simulink model "bh_DBL_CONTROL"  (R2016a)
settings: Solver=ode15s  StartTime=0.0  StopTime=30  FixedStep=0.01  RelTol=1e-5
undefined symbols (not defined in the file or in its folder): b1_damp, b2_damp, g, I1g, I2g, L1x, L2x, mass1, mass2
libraries: simulink x5
settings Model: Creator=bhorton  LastModifiedBy=bhorton
settings SolverCC: ZeroCrossAlgorithm=Adaptive
settings GRTTargetCC: GeneratePreprocessorConditionals=Use local settings
settings SimscapeCC: SimscapeLogType=all  SimscapeLogDataHistory=10000  SelectedTab=Simscape Multibody

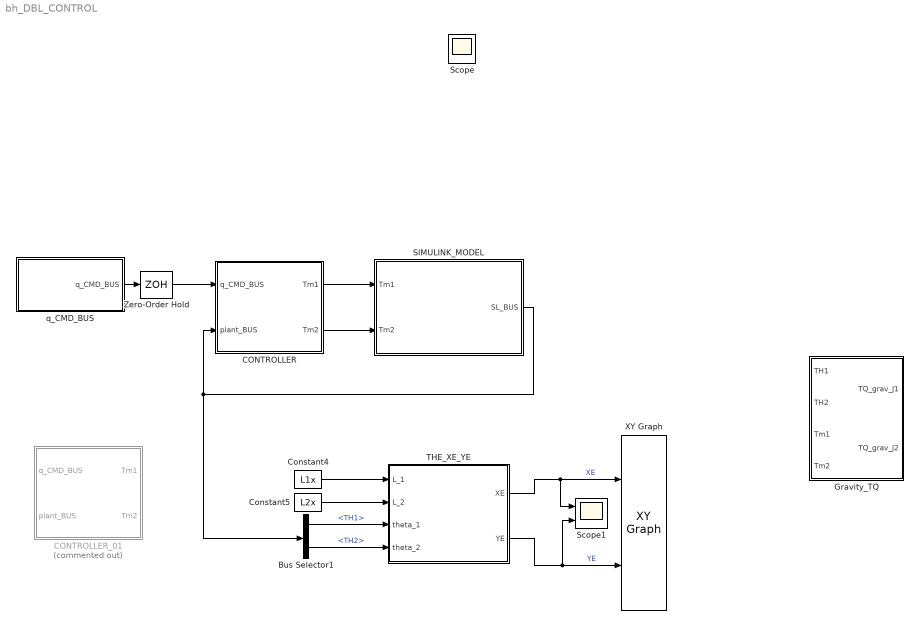
== system bh_DBL_CONTROL ==
  Bus Selector1 : BusSelector  OutputSignals=TH1,TH2
  CONTROLLER : Subsystem
  CONTROLLER_01 : Subsystem  Commented=on
  Constant4 : Constant  Value=L1x
  Constant5 : Constant  Value=L2x
  Gravity_TQ : Subsystem
  SIMULINK_MODEL : Subsystem
  Scope1 : Scope  NumInputPorts=2
  THE_XE_YE : MATLAB Function  TreatAsAtomicUnit=on
  XY Graph : simulink/Sinks/XY Graph  xmin=0  xmax=1.6  ymin=0  ymax=1.6  st=-1
  Zero-Order Hold : ZeroOrderHold  SampleTime=0.01
  q_CMD_BUS : Subsystem
  Scope : Scope
  wires:
  SIMULINK_MODEL/1(SL_BUS) -> CONTROLLER/2(plant_BUS), Bus Selector1/1
  CONTROLLER/1(Tm1) -> SIMULINK_MODEL/1(Tm1)
  CONTROLLER/2(Tm2) -> SIMULINK_MODEL/2(Tm2)
  q_CMD_BUS/1(q_CMD_BUS) -> Zero-Order Hold/1
  Constant5/1 -> THE_XE_YE/2(L_2)
  Constant4/1 -> THE_XE_YE/1(L_1)
  THE_XE_YE/1(XE) -> Scope1/1, XY Graph/1  "XE"
  THE_XE_YE/2(YE) -> Scope1/2, XY Graph/2  "YE"
  Bus Selector1/1 -> THE_XE_YE/3(theta_1)  "<TH1>"
  Bus Selector1/2 -> THE_XE_YE/4(theta_2)  "<TH2>"
  Zero-Order Hold/1 -> CONTROLLER/1(q_CMD_BUS)

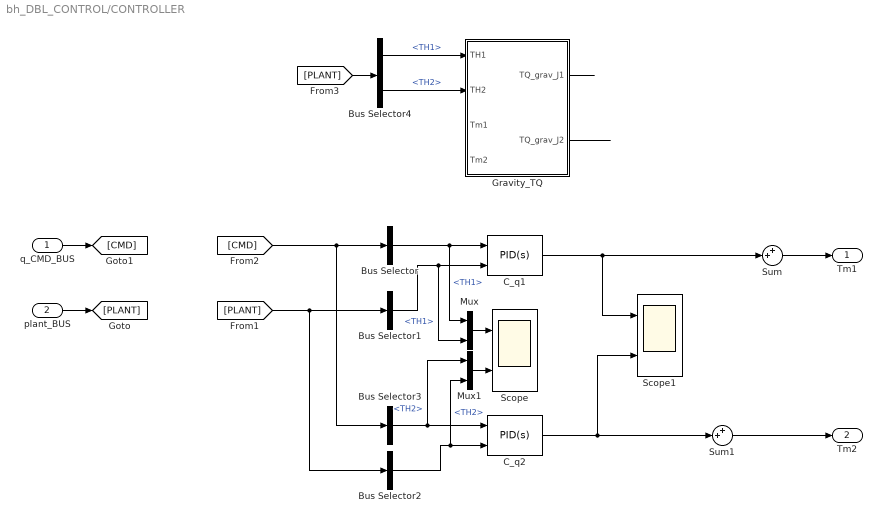
== system bh_DBL_CONTROL/CONTROLLER ==
  q_CMD_BUS : Inport
  plant_BUS : Inport  Port=2
  Bus Selector : BusSelector  OutputSignals=TH1
  Bus Selector1 : BusSelector  OutputSignals=TH1
  Bus Selector2 : BusSelector  OutputSignals=TH2
  Bus Selector3 : BusSelector  OutputSignals=TH2
  Bus Selector4 : BusSelector  OutputSignals=TH1,TH2
  C_q1 : simulink/Continuous/PID Controller (2DOF)  Controller=PID  TimeDomain=Continuous-time  SampleTime=-1  IntegratorMethod=Forward Euler  FilterMethod=Forward Euler  Form=Parallel  UseFilter=on  ControllerParametersSource=internal  P=1357.56511671981  I=4845.84125529163  D=84.5236806608288  N=69907.371435519  b=0.974411131828766  c=0.922736671022408  InitialConditionSource=internal  InitialConditionForIntegrator=0  InitialConditionForFilter=0  ExternalReset=none  LimitOutput=off  UpperSaturationLimit=inf  LowerSaturationLimit=-inf  LinearizeAsGain=on  AntiWindupMode=none  Kb=1  TrackingMode=off  Kt=1  PParamMin=[]  PParamMax=[]  IParamMin=[]  IParamMax=[]  DParamMin=[]  DParamMax=[]  NParamMin=[]  NParamMax=[]  bParamMin=[]  bParamMax=[]  cParamMin=[]  cParamMax=[]  KbParamMin=[]  KbParamMax=[]  KtParamMin=[]  KtParamMax=[]  POutMin=[]  POutMax=[]  IOutMin=[]  IOutMax=[]  DOutMin=[]  DOutMax=[]  NOutMin=[]  NOutMax=[]  bOutMin=[]  bOutMax=[]  cOutMin=[]  cOutMax=[]  KbOutMin=[]  KbOutMax=[]  KtOutMin=[]  KtOutMax=[]  IntegratorOutMin=[]  IntegratorOutMax=[]  FilterOutMin=[]  FilterOutMax=[]  SumOutMin=[]  SumOutMax=[]  Sum1OutMin=[]  Sum1OutMax=[]  Sum2OutMin=[]  Sum2OutMax=[]  Sum3OutMin=[]  Sum3OutMax=[]  SumI1OutMin=[]  SumI1OutMax=[]  SumI2OutMin=[]  SumI2OutMax=[]  SumI3OutMin=[]  SumI3OutMax=[]  SumDOutMin=[]  SumDOutMax=[]  SaturationOutMin=[]  SaturationOutMax=[]  IntegratorContinuousStateAttributes=''  IntegratorStateMustResolveToSignalObject=off  IntegratorRTWStateStorageClass=Auto  FilterContinuousStateAttributes=''  FilterStateMustResolveToSignalObject=off  FilterRTWStateStorageClass=Auto  DifferentiatorICPrevScaledInput=0  DifferentiatorOutMin=[]  DifferentiatorOutMax=[]
  C_q2 : simulink/Continuous/PID Controller (2DOF)  Controller=PID  TimeDomain=Continuous-time  SampleTime=-1  IntegratorMethod=Forward Euler  FilterMethod=Forward Euler  Form=Parallel  UseFilter=on  ControllerParametersSource=internal  P=8716881.64195116  I=38875375820.2039  D=480.022145350049  N=516158.444640812  b=1.01267061686983  c=0.794786207270043  InitialConditionSource=internal  InitialConditionForIntegrator=0  InitialConditionForFilter=0  ExternalReset=none  LimitOutput=off  UpperSaturationLimit=inf  LowerSaturationLimit=-inf  LinearizeAsGain=on  AntiWindupMode=none  Kb=1  TrackingMode=off  Kt=1  PParamMin=[]  PParamMax=[]  IParamMin=[]  IParamMax=[]  DParamMin=[]  DParamMax=[]  NParamMin=[]  NParamMax=[]  bParamMin=[]  bParamMax=[]  cParamMin=[]  cParamMax=[]  KbParamMin=[]  KbParamMax=[]  KtParamMin=[]  KtParamMax=[]  POutMin=[]  POutMax=[]  IOutMin=[]  IOutMax=[]  DOutMin=[]  DOutMax=[]  NOutMin=[]  NOutMax=[]  bOutMin=[]  bOutMax=[]  cOutMin=[]  cOutMax=[]  KbOutMin=[]  KbOutMax=[]  KtOutMin=[]  KtOutMax=[]  IntegratorOutMin=[]  IntegratorOutMax=[]  FilterOutMin=[]  FilterOutMax=[]  SumOutMin=[]  SumOutMax=[]  Sum1OutMin=[]  Sum1OutMax=[]  Sum2OutMin=[]  Sum2OutMax=[]  Sum3OutMin=[]  Sum3OutMax=[]  SumI1OutMin=[]  SumI1OutMax=[]  SumI2OutMin=[]  SumI2OutMax=[]  SumI3OutMin=[]  SumI3OutMax=[]  SumDOutMin=[]  SumDOutMax=[]  SaturationOutMin=[]  SaturationOutMax=[]  IntegratorContinuousStateAttributes=''  IntegratorStateMustResolveToSignalObject=off  IntegratorRTWStateStorageClass=Auto  FilterContinuousStateAttributes=''  FilterStateMustResolveToSignalObject=off  FilterRTWStateStorageClass=Auto  DifferentiatorICPrevScaledInput=0  DifferentiatorOutMin=[]  DifferentiatorOutMax=[]
  Gravity_TQ : Subsystem
  Mux : Mux  Inputs=2
  Mux1 : Mux  Inputs=2
  Scope : Scope  NumInputPorts=2
  Scope1 : Scope  NumInputPorts=2
  Sum : Sum  Inputs=++|
  Sum1 : Sum  Inputs=++|
  Tm1 : Outport
  Tm2 : Outport  Port=2
  wires:
  [CMD] -> Bus Selector3/1, Bus Selector/1
  [PLANT] -> Bus Selector2/1, Bus Selector1/1
  Bus Selector/1 -> Mux/1, C_q1/1  "<TH1>"
  Bus Selector1/1 -> Mux/2, C_q1/2  "<TH1>"
  Bus Selector3/1 -> Mux1/1, C_q2/1  "<TH2>"
  Bus Selector2/1 -> C_q2/2, Mux1/2  "<TH2>"
  Mux/1 -> Scope/1
  Mux1/1 -> Scope/2
  plant_BUS/1 -> [PLANT]
  q_CMD_BUS/1 -> [CMD]
  [PLANT] -> Bus Selector4/1
  Bus Selector4/1 -> Gravity_TQ/1(TH1)  "<TH1>"
  Bus Selector4/2 -> Gravity_TQ/2(TH2)  "<TH2>"
  Sum/1 -> Tm1/1
  C_q1/1 -> Scope1/1, Sum/2
  Gravity_TQ/1(TQ_grav_J1) -> ?
  Gravity_TQ/2(TQ_grav_J2) -> ?
  Sum1/1 -> Tm2/1
  C_q2/1 -> Scope1/2, Sum1/2

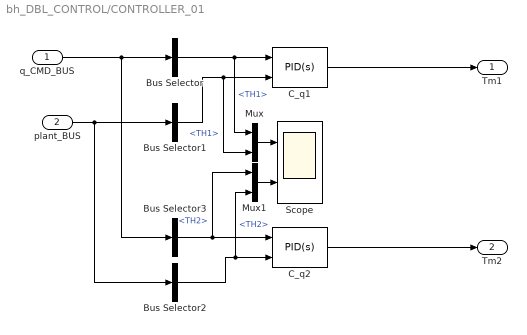
== system bh_DBL_CONTROL/CONTROLLER_01 ==
  q_CMD_BUS : Inport
  plant_BUS : Inport  Port=2
  Bus Selector : BusSelector  OutputSignals=TH1
  Bus Selector1 : BusSelector  OutputSignals=TH1
  Bus Selector2 : BusSelector  OutputSignals=TH2
  Bus Selector3 : BusSelector  OutputSignals=TH2
  C_q1 : simulink/Continuous/PID Controller (2DOF)  Controller=PID  TimeDomain=Continuous-time  SampleTime=-1  IntegratorMethod=Forward Euler  FilterMethod=Forward Euler  Form=Parallel  UseFilter=on  ControllerParametersSource=internal  P=1357.56511671981  I=4845.84125529163  D=84.5236806608288  N=69907.371435519  b=0.974411131828766  c=0.922736671022408  InitialConditionSource=internal  InitialConditionForIntegrator=0  InitialConditionForFilter=0  ExternalReset=none  LimitOutput=off  UpperSaturationLimit=inf  LowerSaturationLimit=-inf  LinearizeAsGain=on  AntiWindupMode=none  Kb=1  TrackingMode=off  Kt=1  PParamMin=[]  PParamMax=[]  IParamMin=[]  IParamMax=[]  DParamMin=[]  DParamMax=[]  NParamMin=[]  NParamMax=[]  bParamMin=[]  bParamMax=[]  cParamMin=[]  cParamMax=[]  KbParamMin=[]  KbParamMax=[]  KtParamMin=[]  KtParamMax=[]  POutMin=[]  POutMax=[]  IOutMin=[]  IOutMax=[]  DOutMin=[]  DOutMax=[]  NOutMin=[]  NOutMax=[]  bOutMin=[]  bOutMax=[]  cOutMin=[]  cOutMax=[]  KbOutMin=[]  KbOutMax=[]  KtOutMin=[]  KtOutMax=[]  IntegratorOutMin=[]  IntegratorOutMax=[]  FilterOutMin=[]  FilterOutMax=[]  SumOutMin=[]  SumOutMax=[]  Sum1OutMin=[]  Sum1OutMax=[]  Sum2OutMin=[]  Sum2OutMax=[]  Sum3OutMin=[]  Sum3OutMax=[]  SumI1OutMin=[]  SumI1OutMax=[]  SumI2OutMin=[]  SumI2OutMax=[]  SumI3OutMin=[]  SumI3OutMax=[]  SumDOutMin=[]  SumDOutMax=[]  SaturationOutMin=[]  SaturationOutMax=[]  IntegratorContinuousStateAttributes=''  IntegratorStateMustResolveToSignalObject=off  IntegratorRTWStateStorageClass=Auto  FilterContinuousStateAttributes=''  FilterStateMustResolveToSignalObject=off  FilterRTWStateStorageClass=Auto  DifferentiatorICPrevScaledInput=0  DifferentiatorOutMin=[]  DifferentiatorOutMax=[]
  C_q2 : simulink/Continuous/PID Controller (2DOF)  Controller=PID  TimeDomain=Continuous-time  SampleTime=-1  IntegratorMethod=Forward Euler  FilterMethod=Forward Euler  Form=Parallel  UseFilter=on  ControllerParametersSource=internal  P=8716881.64195116  I=38875375820.2039  D=480.022145350049  N=516158.444640812  b=1.01267061686983  c=0.794786207270043  InitialConditionSource=internal  InitialConditionForIntegrator=0  InitialConditionForFilter=0  ExternalReset=none  LimitOutput=off  UpperSaturationLimit=inf  LowerSaturationLimit=-inf  LinearizeAsGain=on  AntiWindupMode=none  Kb=1  TrackingMode=off  Kt=1  PParamMin=[]  PParamMax=[]  IParamMin=[]  IParamMax=[]  DParamMin=[]  DParamMax=[]  NParamMin=[]  NParamMax=[]  bParamMin=[]  bParamMax=[]  cParamMin=[]  cParamMax=[]  KbParamMin=[]  KbParamMax=[]  KtParamMin=[]  KtParamMax=[]  POutMin=[]  POutMax=[]  IOutMin=[]  IOutMax=[]  DOutMin=[]  DOutMax=[]  NOutMin=[]  NOutMax=[]  bOutMin=[]  bOutMax=[]  cOutMin=[]  cOutMax=[]  KbOutMin=[]  KbOutMax=[]  KtOutMin=[]  KtOutMax=[]  IntegratorOutMin=[]  IntegratorOutMax=[]  FilterOutMin=[]  FilterOutMax=[]  SumOutMin=[]  SumOutMax=[]  Sum1OutMin=[]  Sum1OutMax=[]  Sum2OutMin=[]  Sum2OutMax=[]  Sum3OutMin=[]  Sum3OutMax=[]  SumI1OutMin=[]  SumI1OutMax=[]  SumI2OutMin=[]  SumI2OutMax=[]  SumI3OutMin=[]  SumI3OutMax=[]  SumDOutMin=[]  SumDOutMax=[]  SaturationOutMin=[]  SaturationOutMax=[]  IntegratorContinuousStateAttributes=''  IntegratorStateMustResolveToSignalObject=off  IntegratorRTWStateStorageClass=Auto  FilterContinuousStateAttributes=''  FilterStateMustResolveToSignalObject=off  FilterRTWStateStorageClass=Auto  DifferentiatorICPrevScaledInput=0  DifferentiatorOutMin=[]  DifferentiatorOutMax=[]
  Mux : Mux  Inputs=2
  Mux1 : Mux  Inputs=2
  Scope : Scope  NumInputPorts=2
  Tm1 : Outport
  Tm2 : Outport  Port=2
  wires:
  q_CMD_BUS/1 -> Bus Selector3/1, Bus Selector/1
  plant_BUS/1 -> Bus Selector2/1, Bus Selector1/1
  Bus Selector/1 -> Mux/1, C_q1/1  "<TH1>"
  Bus Selector1/1 -> Mux/2, C_q1/2  "<TH1>"
  C_q1/1 -> Tm1/1
  Bus Selector3/1 -> Mux1/1, C_q2/1  "<TH2>"
  Bus Selector2/1 -> C_q2/2, Mux1/2  "<TH2>"
  C_q2/1 -> Tm2/1
  Mux/1 -> Scope/1
  Mux1/1 -> Scope/2

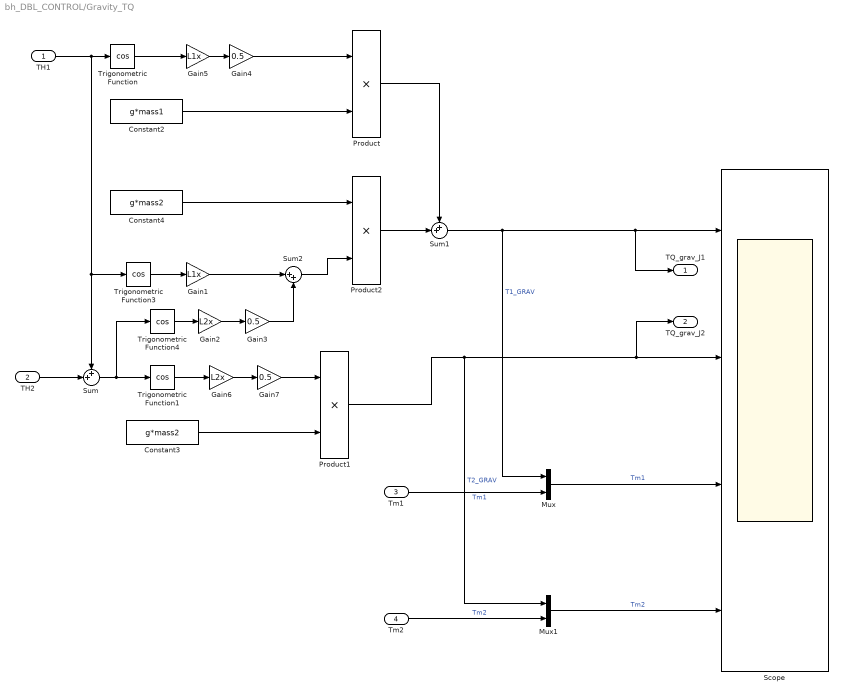
== system bh_DBL_CONTROL/Gravity_TQ ==
  TH1 : Inport
  TH2 : Inport  Port=2
  Tm1 : Inport  Port=3
  Tm2 : Inport  Port=4
  Constant2 : Constant  Value=g*mass1
  Constant3 : Constant  Value=g*mass2
  Constant4 : Constant  Value=g*mass2
  Gain1 : Gain  Gain=L1x
  Gain2 : Gain  Gain=L2x
  Gain3 : Gain  Gain=0.5
  Gain4 : Gain  Gain=0.5
  Gain5 : Gain  Gain=L1x
  Gain6 : Gain  Gain=L2x
  Gain7 : Gain  Gain=0.5
  Mux : Mux  Inputs=2
  Mux1 : Mux  Inputs=2
  Product : Product
  Product1 : Product
  Product2 : Product
  Scope : Scope  NumInputPorts=4
  Sum : Sum  Inputs=++|
  Sum1 : Sum  Inputs=++|
  Sum2 : Sum  Inputs=|++
  Trigonometric Function{,1,3..4} (4 alike) : Trigonometry  Operator=cos
  TQ_grav_J1 : Outport
  TQ_grav_J2 : Outport  Port=2
  wires:
  TH2/1 -> Sum/2
  Sum/1 -> Trigonometric Function4/1, Trigonometric Function1/1
  Trigonometric Function/1 -> Gain5/1
  Trigonometric Function1/1 -> Gain6/1
  Constant3/1 -> Product1/2
  Product/1 -> Sum1/1
  TH1/1 -> Trigonometric Function/1, Trigonometric Function3/1, Sum/1
  Constant2/1 -> Product/2
  Constant4/1 -> Product2/1
  Trigonometric Function3/1 -> Gain1/1
  Gain1/1 -> Sum2/1
  Trigonometric Function4/1 -> Gain2/1
  Gain2/1 -> Gain3/1
  Gain3/1 -> Sum2/2
  Sum2/1 -> Product2/2
  Product2/1 -> Sum1/2
  Sum1/1 -> Mux/1, TQ_grav_J1/1, Scope/1  "T1_GRAV"
  Product1/1 -> Mux1/1, TQ_grav_J2/1, Scope/2  "T2_GRAV"
  Mux/1 -> Scope/3  "Tm1"
  Mux1/1 -> Scope/4  "Tm2"
  Tm1/1 -> Mux/2  "Tm1"
  Tm2/1 -> Mux1/2  "Tm2"
  Gain5/1 -> Gain4/1
  Gain4/1 -> Product/1
  Gain6/1 -> Gain7/1
  Gain7/1 -> Product1/1

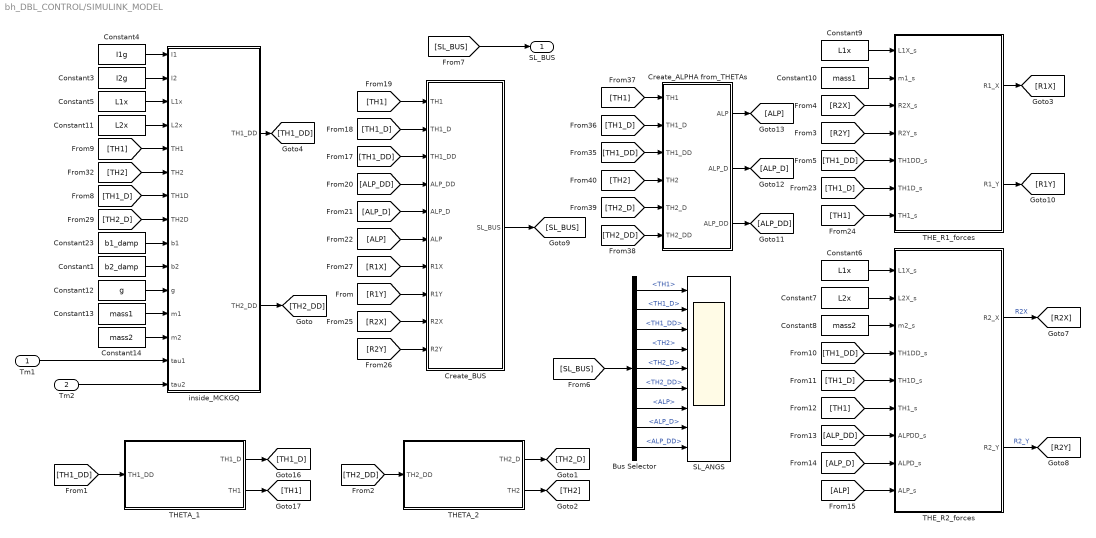
== system bh_DBL_CONTROL/SIMULINK_MODEL ==
  Tm1 : Inport
  Tm2 : Inport  Port=2
  Bus Selector : BusSelector  OutputSignals=TH1,TH1_D,TH1_DD,TH2,TH2_D,TH2_DD,ALP,ALP_D,ALP_DD
  Constant1 : Constant  Value=b2_damp
  Constant10 : Constant  Value=mass1
  Constant11 : Constant  Value=L2x
  Constant12 : Constant  Value=g
  Constant13 : Constant  Value=mass1
  Constant14 : Constant  Value=mass2
  Constant23 : Constant  Value=b1_damp
  Constant3 : Constant  Value=I2g
  Constant4 : Constant  Value=I1g
  Constant5 : Constant  Value=L1x
  Constant6 : Constant  Value=L1x
  Constant7 : Constant  Value=L2x
  Constant8 : Constant  Value=mass2
  Constant9 : Constant  Value=L1x
  Create_ALPHA from_THETAs : Subsystem
  Create_BUS : Subsystem
  SL_ANGS : Scope  NumInputPorts=9
  THETA_1 : Subsystem
  THETA_2 : Subsystem
  THE_R1_forces : MATLAB Function  TreatAsAtomicUnit=on
  THE_R2_forces : MATLAB Function  TreatAsAtomicUnit=on
  inside_MCKGQ : Subsystem
  SL_BUS : Outport
  wires:
  [SL_BUS] -> Bus Selector/1
  [SL_BUS] -> SL_BUS/1
  Constant6/1 -> THE_R2_forces/1(L1X_s)
  Constant7/1 -> THE_R2_forces/2(L2X_s)
  Constant8/1 -> THE_R2_forces/3(m2_s)
  [ALP_DD] -> THE_R2_forces/7(ALPDD_s)
  [ALP_D] -> THE_R2_forces/8(ALPD_s)
  [ALP] -> THE_R2_forces/9(ALP_s)
  [TH1] -> THE_R2_forces/6(TH1_s)
  [TH1_D] -> THE_R2_forces/5(TH1D_s)
  [TH1_DD] -> THE_R2_forces/4(TH1DD_s)
  THE_R2_forces/2(R2_Y) -> [R2Y]  "R2_Y"
  THE_R2_forces/1(R2_X) -> [R2X]  "R2X"
  [ALP_D] -> Create_BUS/5(ALP_D)
  [TH1_D] -> Create_BUS/2(TH1_D)
  [ALP_DD] -> Create_BUS/4(ALP_DD)
  [ALP] -> Create_BUS/6(ALP)
  [TH1_DD] -> Create_BUS/3(TH1_DD)
  [TH1] -> Create_BUS/1(TH1)
  Create_BUS/1(SL_BUS) -> [SL_BUS]
  Bus Selector/2 -> SL_ANGS/2  "<TH1_D>"
  Bus Selector/3 -> SL_ANGS/3  "<TH1_DD>"
  Bus Selector/1 -> SL_ANGS/1  "<TH1>"
  Bus Selector/4 -> SL_ANGS/4  "<TH2>"
  Bus Selector/5 -> SL_ANGS/5  "<TH2_D>"
  Bus Selector/6 -> SL_ANGS/6  "<TH2_DD>"
  Bus Selector/7 -> SL_ANGS/7  "<ALP>"
  Bus Selector/8 -> SL_ANGS/8  "<ALP_D>"
  Bus Selector/9 -> SL_ANGS/9  "<ALP_DD>"
  Constant9/1 -> THE_R1_forces/1(L1X_s)
  Constant10/1 -> THE_R1_forces/2(m1_s)
  [R2X] -> THE_R1_forces/3(R2X_s)
  [R2Y] -> THE_R1_forces/4(R2Y_s)
  [TH1] -> THE_R1_forces/7(TH1_s)
  [TH1_D] -> THE_R1_forces/6(TH1D_s)
  [TH1_DD] -> THE_R1_forces/5(TH1DD_s)
  THE_R1_forces/2(R1_Y) -> [R1Y]
  THE_R1_forces/1(R1_X) -> [R1X]
  [R1X] -> Create_BUS/7(R1X)
  [R1Y] -> Create_BUS/8(R1Y)
  [R2Y] -> Create_BUS/10(R2Y)
  [R2X] -> Create_BUS/9(R2X)
  Constant4/1 -> inside_MCKGQ/1(I1)
  Constant3/1 -> inside_MCKGQ/2(I2)
  Constant11/1 -> inside_MCKGQ/4(L2x)
  Constant5/1 -> inside_MCKGQ/3(L1x)
  Constant12/1 -> inside_MCKGQ/11(g)
  Constant13/1 -> inside_MCKGQ/12(m1)
  Constant14/1 -> inside_MCKGQ/13(m2)
  [TH1] -> inside_MCKGQ/5(TH1)
  [TH2] -> inside_MCKGQ/6(TH2)
  [TH1_D] -> Create_ALPHA from_THETAs/2(TH1_D)
  [TH1_DD] -> Create_ALPHA from_THETAs/3(TH1_DD)
  [TH1] -> Create_ALPHA from_THETAs/1(TH1)
  [TH2] -> Create_ALPHA from_THETAs/4(TH2)
  [TH2_D] -> Create_ALPHA from_THETAs/5(TH2_D)
  [TH2_DD] -> Create_ALPHA from_THETAs/6(TH2_DD)
  Create_ALPHA from_THETAs/2(ALP_D) -> [ALP_D]
  Create_ALPHA from_THETAs/3(ALP_DD) -> [ALP_DD]
  Create_ALPHA from_THETAs/1(ALP) -> [ALP]
  [TH1_D] -> inside_MCKGQ/7(TH1D)
  [TH2_D] -> inside_MCKGQ/8(TH2D)
  [TH2_DD] -> THETA_2/1(TH2_DD)
  THETA_2/2(TH2) -> [TH2]
  THETA_2/1(TH2_D) -> [TH2_D]
  [TH1_DD] -> THETA_1/1(TH1_DD)
  THETA_1/1(TH1_D) -> [TH1_D]
  THETA_1/2(TH1) -> [TH1]
  Constant23/1 -> inside_MCKGQ/9(b1)
  Constant1/1 -> inside_MCKGQ/10(b2)
  inside_MCKGQ/1(TH1_DD) -> [TH1_DD]
  inside_MCKGQ/2(TH2_DD) -> [TH2_DD]
  Tm1/1 -> inside_MCKGQ/14(tau1)
  Tm2/1 -> inside_MCKGQ/15(tau2)

== system bh_DBL_CONTROL/q_CMD_BUS ==
  Bus Creator : BusCreator  Inputs=4
  Bus Selector : BusSelector  OutputSignals=TH1_DOT,TH2_DOT,TH1,TH2
  From Spreadsheet : FromSpreadsheet  FileName=bh_2dof_q1_q2_for_hello.xlsx  SheetName=Q_for_hello  SampleTime=-1  ExtrapolationBeforeFirstDataPoint=Hold first value  ExtrapolationAfterLastDataPoint=Hold last value
  Scope : Scope  NumInputPorts=4
  q_CMD_BUS : Outport
  wires:
  From Spreadsheet/2 -> Bus Creator/2  "TH2_DOT"
  From Spreadsheet/3 -> Bus Creator/3  "TH1"
  From Spreadsheet/1 -> Bus Creator/1  "TH1_DOT"
  From Spreadsheet/4 -> Bus Creator/4  "TH2"
  Bus Creator/1 -> Bus Selector/1, q_CMD_BUS/1
  Bus Selector/1 -> Scope/1  "<TH1_DOT>"
  Bus Selector/2 -> Scope/2  "<TH2_DOT>"
  Bus Selector/3 -> Scope/3  "<TH1>"
  Bus Selector/4 -> Scope/4  "<TH2>"

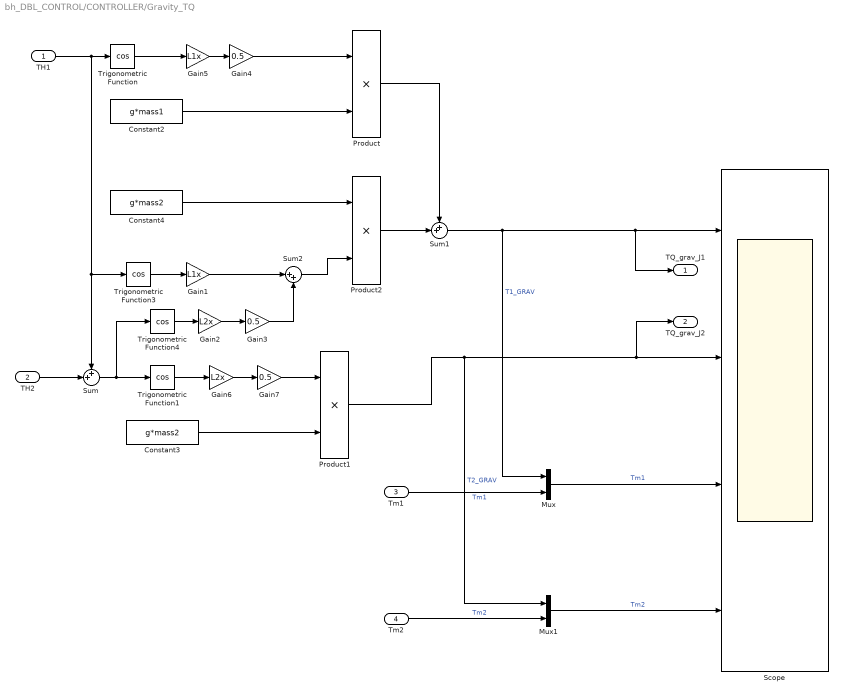
== system bh_DBL_CONTROL/CONTROLLER/Gravity_TQ ==
  TH1 : Inport
  TH2 : Inport  Port=2
  Tm1 : Inport  Port=3
  Tm2 : Inport  Port=4
  Constant2 : Constant  Value=g*mass1
  Constant3 : Constant  Value=g*mass2
  Constant4 : Constant  Value=g*mass2
  Gain1 : Gain  Gain=L1x
  Gain2 : Gain  Gain=L2x
  Gain3 : Gain  Gain=0.5
  Gain4 : Gain  Gain=0.5
  Gain5 : Gain  Gain=L1x
  Gain6 : Gain  Gain=L2x
  Gain7 : Gain  Gain=0.5
  Mux : Mux  Inputs=2
  Mux1 : Mux  Inputs=2
  Product : Product
  Product1 : Product
  Product2 : Product
  Scope : Scope  NumInputPorts=4
  Sum : Sum  Inputs=++|
  Sum1 : Sum  Inputs=++|
  Sum2 : Sum  Inputs=|++
  Trigonometric Function{,1,3..4} (4 alike) : Trigonometry  Operator=cos
  TQ_grav_J1 : Outport
  TQ_grav_J2 : Outport  Port=2
  wires:
  TH2/1 -> Sum/2
  Sum/1 -> Trigonometric Function4/1, Trigonometric Function1/1
  Trigonometric Function/1 -> Gain5/1
  Trigonometric Function1/1 -> Gain6/1
  Constant3/1 -> Product1/2
  Product/1 -> Sum1/1
  TH1/1 -> Trigonometric Function/1, Trigonometric Function3/1, Sum/1
  Constant2/1 -> Product/2
  Constant4/1 -> Product2/1
  Trigonometric Function3/1 -> Gain1/1
  Gain1/1 -> Sum2/1
  Trigonometric Function4/1 -> Gain2/1
  Gain2/1 -> Gain3/1
  Gain3/1 -> Sum2/2
  Sum2/1 -> Product2/2
  Product2/1 -> Sum1/2
  Sum1/1 -> Mux/1, TQ_grav_J1/1, Scope/1  "T1_GRAV"
  Product1/1 -> Mux1/1, TQ_grav_J2/1, Scope/2  "T2_GRAV"
  Mux/1 -> Scope/3  "Tm1"
  Mux1/1 -> Scope/4  "Tm2"
  Tm1/1 -> Mux/2  "Tm1"
  Tm2/1 -> Mux1/2  "Tm2"
  Gain5/1 -> Gain4/1
  Gain4/1 -> Product/1
  Gain6/1 -> Gain7/1
  Gain7/1 -> Product1/1

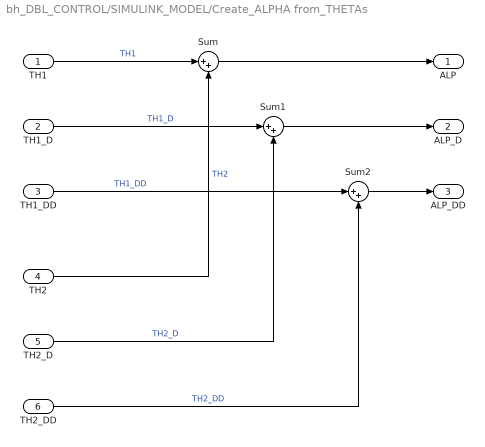
== system bh_DBL_CONTROL/SIMULINK_MODEL/Create_ALPHA from_THETAs ==
  TH1 : Inport
  TH1_D : Inport  Port=2
  TH1_DD : Inport  Port=3
  TH2 : Inport  Port=4
  TH2_D : Inport  Port=5
  TH2_DD : Inport  Port=6
  Sum : Sum  Inputs=|++
  Sum1 : Sum  Inputs=|++
  Sum2 : Sum  Inputs=|++
  ALP : Outport
  ALP_D : Outport  Port=2
  ALP_DD : Outport  Port=3
  wires:
  TH1_DD/1 -> Sum2/1  "TH1_DD"
  TH1_D/1 -> Sum1/1  "TH1_D"
  TH1/1 -> Sum/1  "TH1"
  TH2_DD/1 -> Sum2/2  "TH2_DD"
  TH2_D/1 -> Sum1/2  "TH2_D"
  TH2/1 -> Sum/2  "TH2"
  Sum/1 -> ALP/1
  Sum1/1 -> ALP_D/1
  Sum2/1 -> ALP_DD/1

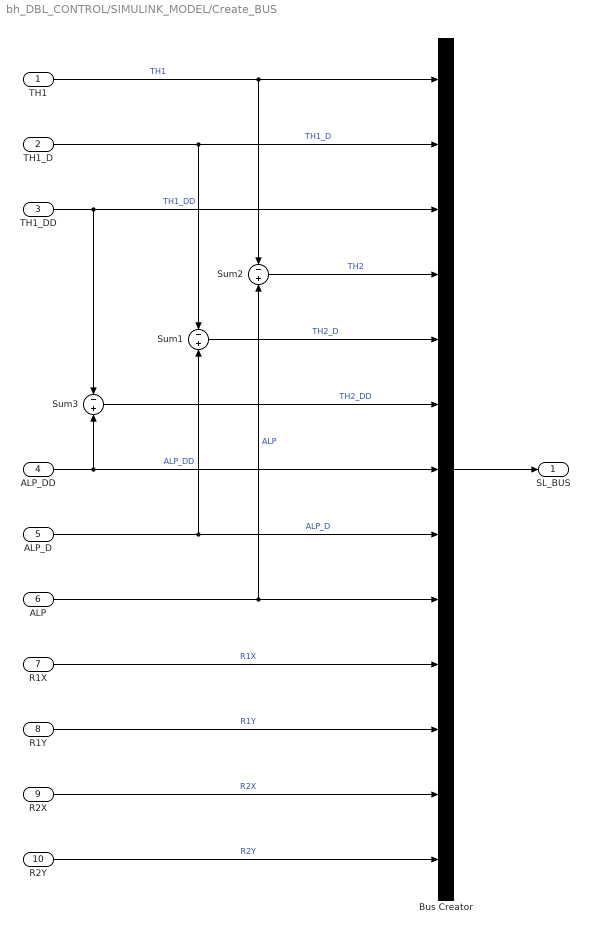
== system bh_DBL_CONTROL/SIMULINK_MODEL/Create_BUS ==
  TH1 : Inport
  TH1_D : Inport  Port=2
  TH1_DD : Inport  Port=3
  ALP_DD : Inport  Port=4
  ALP_D : Inport  Port=5
  ALP : Inport  Port=6
  R1X : Inport  Port=7
  R1Y : Inport  Port=8
  R2X : Inport  Port=9
  R2Y : Inport  Port=10
  Bus Creator : BusCreator  Inputs=13
  Sum1 : Sum  Inputs=-|+
  Sum2 : Sum  Inputs=-|+
  Sum3 : Sum  Inputs=-|+
  SL_BUS : Outport
  wires:
  ALP_DD/1 -> Bus Creator/7, Sum3/2  "ALP_DD"
  TH1_DD/1 -> Sum3/1, Bus Creator/3  "TH1_DD"
  TH1_D/1 -> Bus Creator/2, Sum1/1  "TH1_D"
  ALP_D/1 -> Bus Creator/8, Sum1/2  "ALP_D"
  TH1/1 -> Bus Creator/1, Sum2/1  "TH1"
  ALP/1 -> Bus Creator/9, Sum2/2  "ALP"
  Sum2/1 -> Bus Creator/4  "TH2"
  Sum1/1 -> Bus Creator/5  "TH2_D"
  Sum3/1 -> Bus Creator/6  "TH2_DD"
  Bus Creator/1 -> SL_BUS/1
  R1Y/1 -> Bus Creator/11  "R1Y"
  R1X/1 -> Bus Creator/10  "R1X"
  R2Y/1 -> Bus Creator/13  "R2Y"
  R2X/1 -> Bus Creator/12  "R2X"

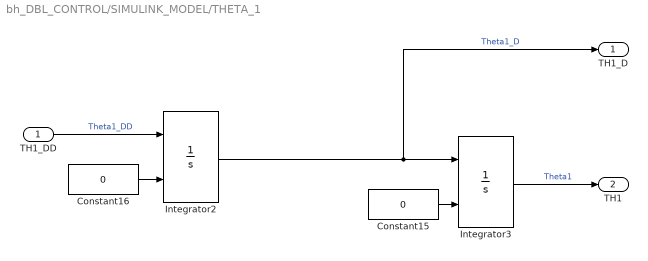
== system bh_DBL_CONTROL/SIMULINK_MODEL/THETA_1 ==
  TH1_DD : Inport
  Constant15 : Constant  Value=0
  Constant16 : Constant  Value=0
  Integrator2 : Integrator  InitialConditionSource=external
  Integrator3 : Integrator  InitialConditionSource=external
  TH1_D : Outport
  TH1 : Outport  Port=2
  wires:
  TH1_DD/1 -> Integrator2/1  "Theta1_DD"
  Constant15/1 -> Integrator3/2
  Constant16/1 -> Integrator2/2
  Integrator3/1 -> TH1/1  "Theta1"
  Integrator2/1 -> TH1_D/1, Integrator3/1  "Theta1_D"

== system bh_DBL_CONTROL/SIMULINK_MODEL/THETA_2 ==
  TH2_DD : Inport
  Constant15 : Constant  Value=0
  Constant16 : Constant  Value=0
  Integrator2 : Integrator  InitialConditionSource=external
  Integrator3 : Integrator  InitialConditionSource=external
  TH2_D : Outport
  TH2 : Outport  Port=2
  wires:
  TH2_DD/1 -> Integrator2/1  "Theta2_DD"
  Integrator2/1 -> TH2_D/1, Integrator3/1  "Theta2_D"
  Constant15/1 -> Integrator3/2
  Constant16/1 -> Integrator2/2
  Integrator3/1 -> TH2/1  "Theta2"

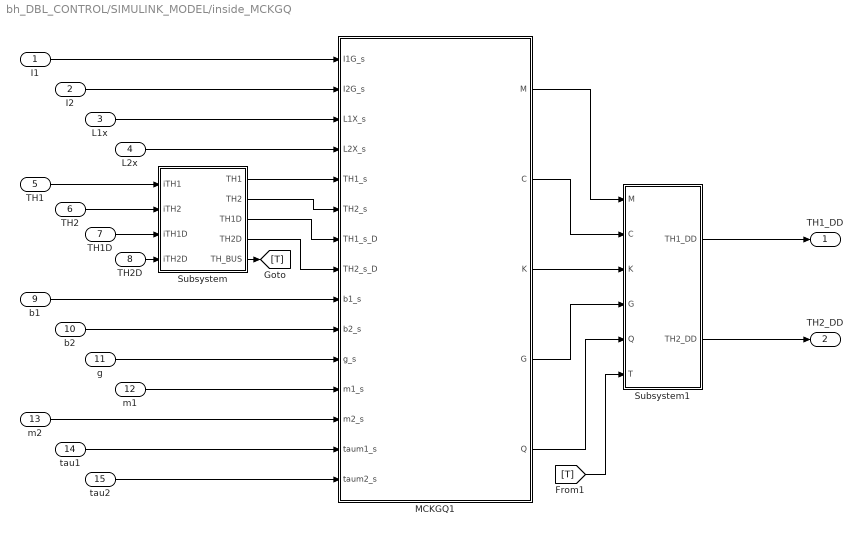
== system bh_DBL_CONTROL/SIMULINK_MODEL/inside_MCKGQ ==
  I1 : Inport
  I2 : Inport  Port=2
  L1x : Inport  Port=3
  L2x : Inport  Port=4
  TH1 : Inport  Port=5
  TH2 : Inport  Port=6
  TH1D : Inport  Port=7
  TH2D : Inport  Port=8
  b1 : Inport  Port=9
  b2 : Inport  Port=10
  g : Inport  Port=11
  m1 : Inport  Port=12
  m2 : Inport  Port=13
  tau1 : Inport  Port=14
  tau2 : Inport  Port=15
  MCKGQ1 : MATLAB Function  TreatAsAtomicUnit=on
  Subsystem : Subsystem
  Subsystem1 : Subsystem
  TH1_DD : Outport
  TH2_DD : Outport  Port=2
  wires:
  I1/1 -> MCKGQ1/1(I1G_s)
  m2/1 -> MCKGQ1/13(m2_s)
  b2/1 -> MCKGQ1/10(b2_s)
  L2x/1 -> MCKGQ1/4(L2X_s)
  m1/1 -> MCKGQ1/12(m1_s)
  L1x/1 -> MCKGQ1/3(L1X_s)
  b1/1 -> MCKGQ1/9(b1_s)
  tau2/1 -> MCKGQ1/15(taum2_s)
  tau1/1 -> MCKGQ1/14(taum1_s)
  g/1 -> MCKGQ1/11(g_s)
  I2/1 -> MCKGQ1/2(I2G_s)
  Subsystem/2(TH2) -> MCKGQ1/6(TH2_s)
  Subsystem/1(TH1) -> MCKGQ1/5(TH1_s)
  Subsystem/3(TH1D) -> MCKGQ1/7(TH1_s_D)
  Subsystem/4(TH2D) -> MCKGQ1/8(TH2_s_D)
  TH2D/1 -> Subsystem/4(iTH2D)
  TH1D/1 -> Subsystem/3(iTH1D)
  TH2/1 -> Subsystem/2(iTH2)
  TH1/1 -> Subsystem/1(iTH1)
  Subsystem/5(TH_BUS) -> [T]
  [T] -> Subsystem1/6(T)
  MCKGQ1/3(K) -> Subsystem1/3(K)
  MCKGQ1/4(G) -> Subsystem1/4(G)
  MCKGQ1/5(Q) -> Subsystem1/5(Q)
  MCKGQ1/2(C) -> Subsystem1/2(C)
  MCKGQ1/1(M) -> Subsystem1/1(M)
  Subsystem1/1(TH1_DD) -> TH1_DD/1
  Subsystem1/2(TH2_DD) -> TH2_DD/1

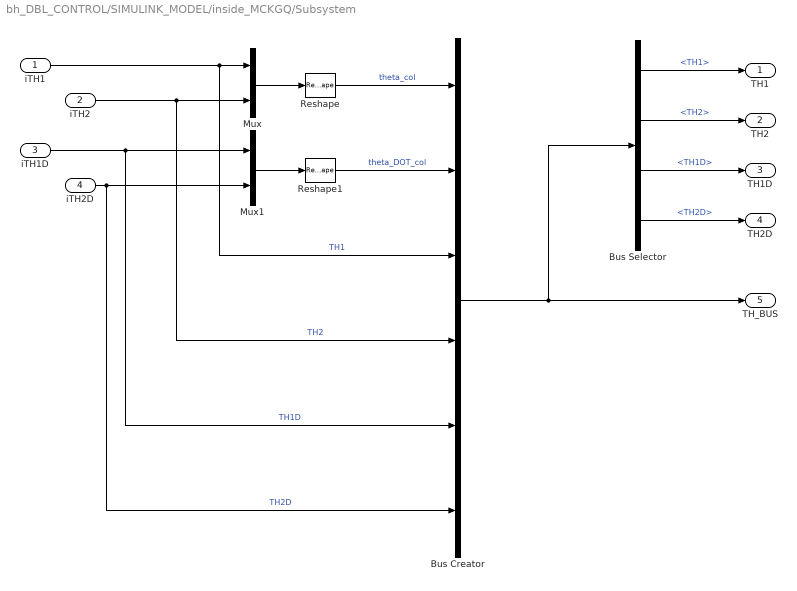
== system bh_DBL_CONTROL/SIMULINK_MODEL/inside_MCKGQ/Subsystem ==
  iTH1 : Inport
  iTH2 : Inport  Port=2
  iTH1D : Inport  Port=3
  iTH2D : Inport  Port=4
  Bus Creator : BusCreator  Inputs=6
  Bus Selector : BusSelector  OutputSignals=TH1,TH2,TH1D,TH2D
  Mux : Mux  Inputs=2
  Mux1 : Mux  Inputs=2
  Reshape : Reshape  OutputDimensionality=Column vector (2-D)
  Reshape1 : Reshape  OutputDimensionality=Column vector (2-D)
  TH1 : Outport
  TH2 : Outport  Port=2
  TH1D : Outport  Port=3
  TH2D : Outport  Port=4
  TH_BUS : Outport  Port=5
  wires:
  iTH2/1 -> Bus Creator/4, Mux/2  "TH2"
  iTH1/1 -> Bus Creator/3, Mux/1  "TH1"
  iTH2D/1 -> Bus Creator/6, Mux1/2  "TH2D"
  iTH1D/1 -> Bus Creator/5, Mux1/1  "TH1D"
  Mux/1 -> Reshape/1
  Mux1/1 -> Reshape1/1
  Reshape/1 -> Bus Creator/1  "theta_col"
  Reshape1/1 -> Bus Creator/2  "theta_DOT_col"
  Bus Creator/1 -> Bus Selector/1, TH_BUS/1
  Bus Selector/1 -> TH1/1  "<TH1>"
  Bus Selector/2 -> TH2/1  "<TH2>"
  Bus Selector/3 -> TH1D/1  "<TH1D>"
  Bus Selector/4 -> TH2D/1  "<TH2D>"

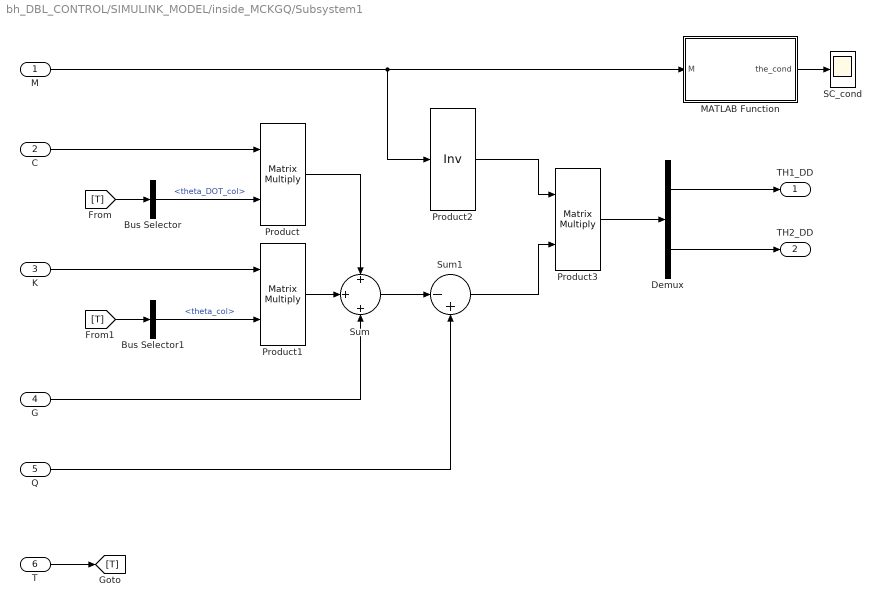
== system bh_DBL_CONTROL/SIMULINK_MODEL/inside_MCKGQ/Subsystem1 ==
  M : Inport
  C : Inport  Port=2
  K : Inport  Port=3
  G : Inport  Port=4
  Q : Inport  Port=5
  T : Inport  Port=6
  Bus Selector : BusSelector  OutputSignals=theta_DOT_col
  Bus Selector1 : BusSelector  OutputSignals=theta_col
  Demux : Demux  Outputs=2
  MATLAB Function : MATLAB Function  TreatAsAtomicUnit=on
  Product : Product  Multiplication=Matrix(*)
  Product1 : Product  Multiplication=Matrix(*)
  Product2 : Product  Inputs=/  Multiplication=Matrix(*)
  Product3 : Product  Multiplication=Matrix(*)
  SC_cond : Scope
  Sum : Sum  Inputs=+|+|+
  Sum1 : Sum  Inputs=|-+
  TH1_DD : Outport
  TH2_DD : Outport  Port=2
  wires:
  T/1 -> [T]
  C/1 -> Product/1
  [T] -> Bus Selector/1
  Bus Selector/1 -> Product/2  "<theta_DOT_col>"
  K/1 -> Product1/1
  [T] -> Bus Selector1/1
  Bus Selector1/1 -> Product1/2  "<theta_col>"
  Q/1 -> Sum1/2
  Product1/1 -> Sum/2
  G/1 -> Sum/3
  Product/1 -> Sum/1
  Sum/1 -> Sum1/1
  M/1 -> Product2/1, MATLAB Function/1(M)
  Product2/1 -> Product3/1
  Sum1/1 -> Product3/2
  Product3/1 -> Demux/1
  Demux/1 -> TH1_DD/1
  Demux/2 -> TH2_DD/1
  MATLAB Function/1(the_cond) -> SC_cond/1

== matlab function bh_DBL_CONTROL/SIMULINK_MODEL/inside_MCKGQ/Subsystem1/MATLAB Function ==
  data: M input; the_cond output
function the_cond = COND(M)
%#codegen

the_cond = cond(M);

end

== matlab function bh_DBL_CONTROL/SIMULINK_MODEL/inside_MCKGQ/MCKGQ1 ==
  data: I1G_s input; M output; I2G_s input; L1X_s input; L2X_s input; TH1_s input; TH2_s input; TH1_s_D input; TH2_s_D input; b1_s input; b2_s input; g_s input; m1_s input; m2_s input; taum1_s input; taum2_s input; C output; K output; G output; Q output
function [M,C,K,G,Q] = MCKGQ(I1G_s,I2G_s,L1X_s,L2X_s,TH1_s,TH2_s,TH1_s_D,TH2_s_D,b1_s,b2_s,g_s,m1_s,m2_s,taum1_s,taum2_s)
%#codegen

%    This function was generated by the Symbolic Math Toolbox version 7.0.
%    09-Sep-2016 14:36:22

M = reshape([I1G_s+I2G_s+L1X_s.^2.*m1_s.*(1.0./4.0)+L1X_s.^2.*m2_s+L2X_s.^2.*m2_s.*(1.0./4.0)+L1X_s.*L2X_s.*m2_s.*cos(TH2_s),I2G_s+L2X_s.^2.*m2_s.*(1.0./4.0)+L1X_s.*L2X_s.*m2_s.*cos(TH2_s).*(1.0./2.0),I2G_s+L2X_s.^2.*m2_s.*(1.0./4.0)+L1X_s.*L2X_s.*m2_s.*cos(TH2_s).*(1.0./2.0),I2G_s+L2X_s.^2.*m2_s.*(1.0./4.0)],[2,2]);
if nargout > 1
    C = reshape([-L1X_s.*L2X_s.*TH2_s_D.*m2_s.*sin(TH2_s),L1X_s.*L2X_s.*TH1_s_D.*m2_s.*sin(TH2_s).*(1.0./2.0),L1X_s.*L2X_s.*TH2_s_D.*m2_s.*sin(TH2_s).*(-1.0./2.0),0.0],[2,2]);
end
if nargout > 2
    K = reshape([0.0,0.0,0.0,0.0],[2,2]);
end
if nargout > 3
    G = [g_s.*(L2X_s.*m2_s.*cos(TH1_s+TH2_s)+L1X_s.*m1_s.*cos(TH1_s)+L1X_s.*m2_s.*cos(TH1_s).*2.0).*(1.0./2.0);L2X_s.*g_s.*m2_s.*cos(TH1_s+TH2_s).*(1.0./2.0)];
end
if nargout > 4
    Q = [taum1_s-TH1_s_D.*b1_s;taum2_s-TH2_s_D.*b2_s];
end

== matlab function bh_DBL_CONTROL/SIMULINK_MODEL/THE_R1_forces ==
  data: L1X_s input; R1_X output; m1_s input; R2X_s input; R2Y_s input; TH1DD_s input; TH1D_s input; TH1_s input; R1_Y output
function [R1_X,R1_Y] = THE_R1_forces(L1X_s,m1_s,R2X_s,R2Y_s,TH1DD_s,TH1D_s,TH1_s)
%#codegen

%    This function was generated by the Symbolic Math Toolbox version 7.0.
%    17-Aug-2016 17:09:15

R1_X = R2X_s-m1_s.*(L1X_s.*TH1D_s.^2.*cos(TH1_s).*(1.0./2.0)+L1X_s.*TH1DD_s.*sin(TH1_s).*(1.0./2.0));
if nargout > 1
    R1_Y = R2Y_s+m1_s.*(9.81e2./1.0e2)-m1_s.*(L1X_s.*TH1D_s.^2.*sin(TH1_s).*(1.0./2.0)-L1X_s.*TH1DD_s.*cos(TH1_s).*(1.0./2.0));
end

== matlab function bh_DBL_CONTROL/SIMULINK_MODEL/THE_R2_forces ==
  data: L1X_s input; R2_X output; L2X_s input; m2_s input; TH1DD_s input; TH1D_s input; TH1_s input; ALPDD_s input; ALPD_s input; ALP_s input; R2_Y output
function [R2_X,R2_Y] = THE_R2_forces(L1X_s,L2X_s,m2_s,TH1DD_s,TH1D_s,TH1_s,ALPDD_s,ALPD_s,ALP_s)
%#codegen

%    This function was generated by the Symbolic Math Toolbox version 7.0.
%    17-Aug-2016 17:09:15

R2_X = -m2_s.*(L1X_s.*TH1D_s.^2.*cos(TH1_s)+ALPDD_s.*L2X_s.*sin(ALP_s).*(1.0./2.0)+L1X_s.*TH1DD_s.*sin(TH1_s)+ALPD_s.^2.*L2X_s.*cos(ALP_s).*(1.0./2.0));
if nargout > 1
    R2_Y = m2_s.*(9.81e2./1.0e2)-m2_s.*(ALPD_s.^2.*L2X_s.*sin(ALP_s).*(1.0./2.0)+L1X_s.*TH1D_s.^2.*sin(TH1_s)-ALPDD_s.*L2X_s.*cos(ALP_s).*(1.0./2.0)-L1X_s.*TH1DD_s.*cos(TH1_s));
end

== matlab function bh_DBL_CONTROL/THE_XE_YE ==
  data: L_1 input; XE output; L_2 input; theta_1 input; theta_2 input; YE output
function [XE,YE] = THE_XEYE(L_1,L_2,theta_1,theta_2)
%#codegen

%    This function was generated by the Symbolic Math Toolbox version 7.0.
%    05-Sep-2016 11:23:53

XE = L_2.*cos(theta_1+theta_2)+L_1.*cos(theta_1);
if nargout > 1
    YE = L_2.*sin(theta_1+theta_2)+L_1.*sin(theta_1);
end
